simulink model "verify_WindowWithShading_Ug_mdl"  (R2016b)
settings: Solver=ode45  StartTime=0  StopTime=6*3600  MaxStep=100  RelTol=1e-3  EnableMultiTasking=on
undefined symbols (not defined in the file or in its folder): Dreifach, Wärmeschutzglas
libraries: carnot x5
settings Model: Creator=drhf  LastModifiedBy=drhf
settings DataIOCC: SaveFormat=Array  SignalLoggingSaveFormat=ModelDataLogs
settings OptimizationCC: ExpressionDepthLimit=2147483647  LifeSpan=inf
settings DebuggingCC: UnderspecifiedInitializationDetection=Classic  MergeDetectMultiDrivingBlocksExec=none  SolverPrmCheckMsg=warning  FcnCallInpInsideContextMsg=warning  StateNameClashWarn=warning  SFUnexpectedBacktrackingDiag=warning  SFNoUnconditionalDefaultTransitionDiag=warning  SFExecutionAtInitializationDiag=none
settings HardwareCC: ProdBitPerPointer=32  ProdBitPerSizeT=32  ProdBitPerPtrDiffT=32  ProdLargestAtomicFloat=None  ProdIntDivRoundTo=Undefined  ProdEndianess=Unspecified  ProdWordSize=32  ProdHWDeviceType=32-bit Generic
settings ModelReferenceCC: PropagateSignalLabelsOutOfModel=off
settings GRTTargetCC: TargetLangStandard=C89/C90 (ANSI)  GeneratePreprocessorConditionals=Disable all  CombineOutputUpdateFcns=off  GRTInterface=on
settings ConfigComp: CovMetricSettings=dw  CovHtmlReporting=on  CovSaveCumulativeToWorkspaceVar=on  CovSaveSingleToWorkspaceVar=on  CovExternalEMLEnable=off

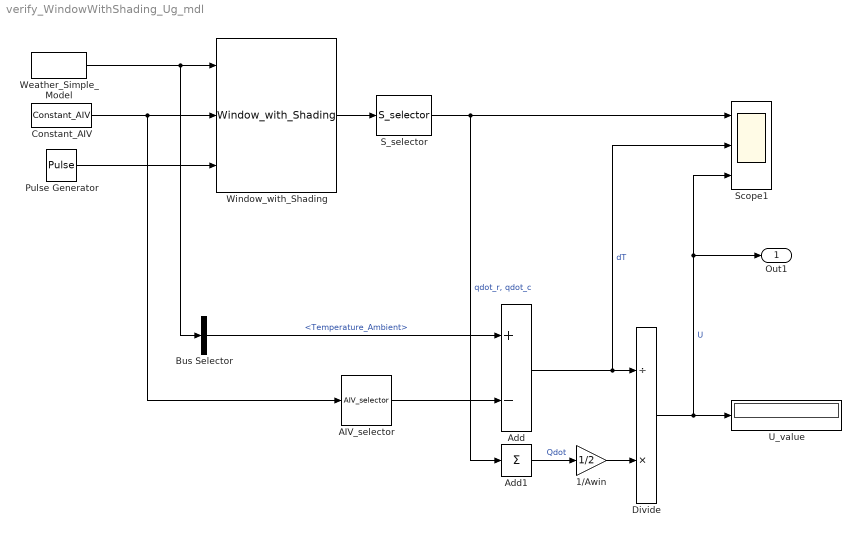
== system verify_WindowWithShading_Ug_mdl ==
  1/Awin : Gain  Gain=1/2
  AIV_selector : carnot/Outputs/AIV_selector  e1=on  e2=off  e3=off  e4=off  e5=off  e6=off  e7=off  e8=off  e9=off
  Add : Sum  Inputs=+-
  Add1 : Sum  Inputs=1
  Bus Selector : BusSelector  OutputSignals=Temperature_Ambient
  Constant_AIV : carnot/Source/Ventilation/Constant_AIV  Tsens=20  Tcon=20  Trad=20  mw=0.012  mco=0.01  rhoair=1.2  cpair=1004  pair=100000  nair=0.5
  Divide : Product  Inputs=/*
  Pulse Generator : DiscretePulseGenerator  PulseType=Time based  Period=3600  PulseWidth=50
  S_selector : carnot/Outputs/S_selector  e1=off  e2=off  e3=off  e4=off  e5=off  e6=off  e7=on  e8=on  e9=off  e10=off  e11=off  e12=off  e13=off
  Scope1 : Scope  NumInputPorts=3
  U_value : Display
  Weather_Simple_Model : carnot/Weather/Weather_Simple_Model  lat=60  Ibn=0  Idg=0  tamb=0  deltaTsky=0  rh=50  precip="10e-3/24/3600           % 10 mm in 24 h"  cloud=0.125  p=1013e2  vw=5.85  wdir=270
  Window_with_Shading : carnot/Load/Houses/wall_floor/Window_with_Shading  pos=180  windowsize=[1 2]  frame=0.1  Ug=1  gvalue=0.7  tauzero=0.8  numpanes=2  d=[0.004 0.004]  rho=[2500 2500]  cp="[1008  1008]"  t0=20  misc="[0.2,  0.1,  1,  1]"  shad_type=No shading  type_glazing=Dreifach-Wärmeschutzglas  tau_shad=0.01  bli_a=0.05  bli_b=1  bli_c=0.05  bli_d=0.05  bli_alpha=90  bli_refl=0.2
  Out1 : Outport
  wires:
  Window_with_Shading/1 -> S_selector/1
  Pulse Generator/1 -> Window_with_Shading/3
  Constant_AIV/1 -> Window_with_Shading/2, AIV_selector/1
  AIV_selector/1 -> Add/2
  Add/1 -> Scope1/2, Divide/1  "dT"
  S_selector/1 -> Add1/1, Scope1/1  "qdot_r, qdot_c"
  Add1/1 -> 1/Awin/1  "Qdot"
  Divide/1 -> U_value/1, Scope1/3, Out1/1  "U"
  Weather_Simple_Model/1 -> Bus Selector/1, Window_with_Shading/1
  Bus Selector/1 -> Add/1  "<Temperature_Ambient>"
  1/Awin/1 -> Divide/2
